simulink model "shr26df_quick_edit"  (R2024b)
settings: Solver=VariableStepAuto  StartTime=0.0  StopTime=2.0  RelTol=1e-3
undefined symbols (not defined in the file): X, Y, Z
libraries: sm_lib x261, nesl_utility x53
(part 1 of 6)
settings Model: Creator=danie  LastModifiedBy=danie

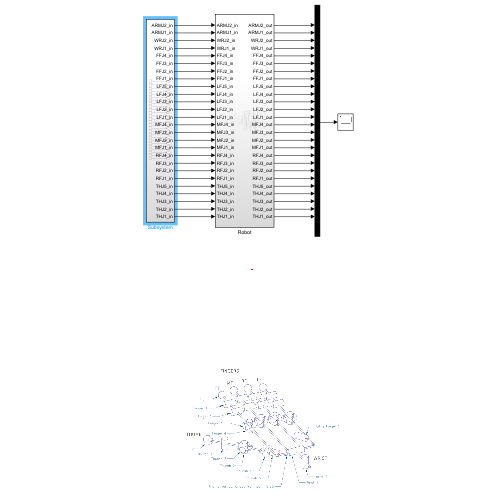
[thumbnail: Simulink's stored preview of the top-level diagram]
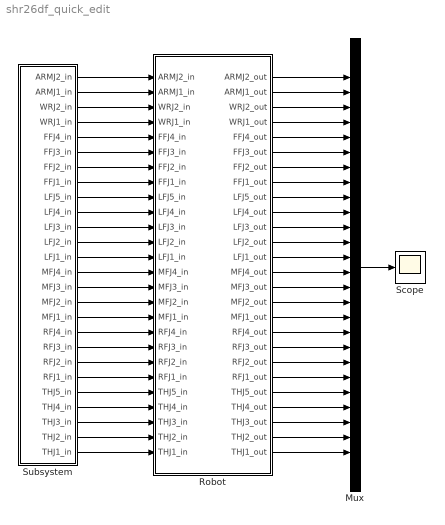
== system shr26df_quick_edit ==
  Mux : Mux  Inputs=26
  Robot : Subsystem
  Scope : Scope
  Subsystem : Subsystem
  wires:
  Mux/1 -> Scope/1
  Subsystem/3(WRJ2_in) -> Robot/3(WRJ2_in)
  Subsystem/4(WRJ1_in) -> Robot/4(WRJ1_in)
  Subsystem/5(FFJ4_in) -> Robot/5(FFJ4_in)
  Subsystem/6(FFJ3_in) -> Robot/6(FFJ3_in)
  Subsystem/7(FFJ2_in) -> Robot/7(FFJ2_in)
  Subsystem/8(FFJ1_in) -> Robot/8(FFJ1_in)
  Subsystem/9(LFJ5_in) -> Robot/9(LFJ5_in)
  Subsystem/10(LFJ4_in) -> Robot/10(LFJ4_in)
  Subsystem/11(LFJ3_in) -> Robot/11(LFJ3_in)
  Subsystem/12(LFJ2_in) -> Robot/12(LFJ2_in)
  Subsystem/13(LFJ1_in) -> Robot/13(LFJ1_in)
  Subsystem/14(MFJ4_in) -> Robot/14(MFJ4_in)
  Subsystem/15(MFJ3_in) -> Robot/15(MFJ3_in)
  Subsystem/16(MFJ2_in) -> Robot/16(MFJ2_in)
  Subsystem/17(MFJ1_in) -> Robot/17(MFJ1_in)
  Subsystem/18(RFJ4_in) -> Robot/18(RFJ4_in)
  Subsystem/19(RFJ3_in) -> Robot/19(RFJ3_in)
  Subsystem/20(RFJ2_in) -> Robot/20(RFJ2_in)
  Subsystem/21(RFJ1_in) -> Robot/21(RFJ1_in)
  Subsystem/22(THJ5_in) -> Robot/22(THJ5_in)
  Subsystem/23(THJ4_in) -> Robot/23(THJ4_in)
  Subsystem/24(THJ3_in) -> Robot/24(THJ3_in)
  Subsystem/25(THJ2_in) -> Robot/25(THJ2_in)
  Subsystem/26(THJ1_in) -> Robot/26(THJ1_in)
  Subsystem/2(ARMJ1_in) -> Robot/2(ARMJ1_in)
  Subsystem/1(ARMJ2_in) -> Robot/1(ARMJ2_in)
  Robot/1(ARMJ2_out) -> Mux/1
  Robot/2(ARMJ1_out) -> Mux/2
  Robot/3(WRJ2_out) -> Mux/3
  Robot/4(WRJ1_out) -> Mux/4
  Robot/5(FFJ4_out) -> Mux/5
  Robot/6(FFJ3_out) -> Mux/6
  Robot/7(FFJ2_out) -> Mux/7
  Robot/8(FFJ1_out) -> Mux/8
  Robot/9(LFJ5_out) -> Mux/9
  Robot/10(LFJ4_out) -> Mux/10
  Robot/11(LFJ3_out) -> Mux/11
  Robot/12(LFJ2_out) -> Mux/12
  Robot/13(LFJ1_out) -> Mux/13
  Robot/14(MFJ4_out) -> Mux/14
  Robot/15(MFJ3_out) -> Mux/15
  Robot/16(MFJ2_out) -> Mux/16
  Robot/17(MFJ1_out) -> Mux/17
  Robot/18(RFJ4_out) -> Mux/18
  Robot/19(RFJ3_out) -> Mux/19
  Robot/20(RFJ2_out) -> Mux/20
  Robot/21(RFJ1_out) -> Mux/21
  Robot/22(THJ5_out) -> Mux/22
  Robot/23(THJ4_out) -> Mux/23
  Robot/24(THJ3_out) -> Mux/24
  Robot/25(THJ2_out) -> Mux/25
  Robot/26(THJ1_out) -> Mux/26
